simulink model "modell_kalman"  (R2013a)
settings: Solver=ode45  SolverMode=SingleTasking  StartTime=0.0  StopTime=10.0  RelTol=1e-3
values from neighbouring files (symbols this model uses):
  A = [0 1 0 0; d3 0 0 0;0 0 0 1; c3 0 0 0]    [startModell.m]
  B = [0 ; d1; 0 ; c1]    [startModell.m]
  beobachterNull = [0;0;0;0]    [startModell.m]
  C = [1 0 0 0; 0 0 1 0]    [startModell.m]
  K = lqr(A,B,Q_ctrl,R_ctrl)    [startModell.m]
  modellNull = [10/180*pi;0;0;0]    [startModell.m]
  P0 = diag([100,100,1,1])    [startModell.m]
  Q = eye(4)    [startModell.m]
  R = diag([10, 10])    [startModell.m]
  Rinv = inv(R)    [startModell.m]
undefined symbols (not defined in the file or in its folder): Filter, Kalman, library
libraries: simulink x1
settings Model: Creator=wall  LastModifiedBy=timoe
settings DataIOCC: SignalLoggingSaveFormat=ModelDataLogs
settings OptimizationCC: BlockReduction=off  BooleanDataType=off
settings DebuggingCC: SaveWithParameterizedLinksMsg=none  SignalResolutionControl=TryResolveAllWithWarning  SolverPrmCheckMsg=none  MultiTaskDSMMsg=warning  MultiTaskCondExecSysMsg=none  StrictBusMsg=None
settings HardwareCC: TargetUnknown=on
settings RTWCC: IncludeERTFirstTime=on

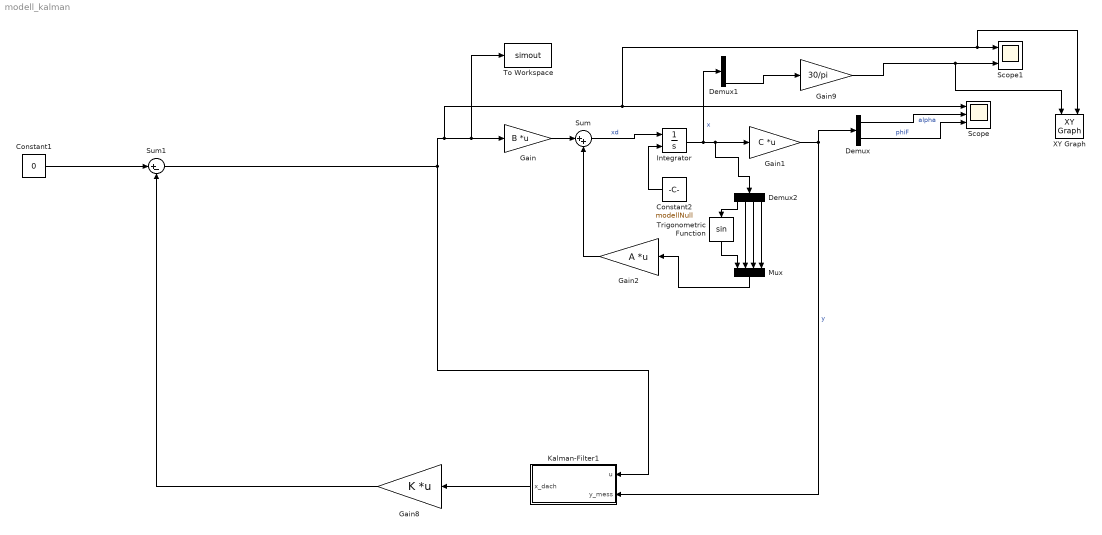
== system modell_kalman ==
  Constant1 : Constant  Value=0
  Constant2 : Constant  Value=modellNull
  Demux : Demux  Outputs=2
  Demux1 : Demux
  Demux2 : Demux
  Gain : Gain  Gain=B  Multiplication=Matrix(K*u) (u vector)
  Gain1 : Gain  Gain=C  Multiplication=Matrix(K*u) (u vector)
  Gain2 : Gain  Gain=A  Multiplication=Matrix(K*u) (u vector)
  Gain8 : Gain  Gain=K  Multiplication=Matrix(K*u) (u vector)
  Gain9 : Gain  Gain=30/pi
  Integrator : Integrator  InitialConditionSource=external
  Kalman-Filter1 : Subsystem  AncestorBlock=library/Kalman-Filter
  Mux : Mux
  Scope : Scope  NumInputPorts=3
      settings: YMin=-1~0.165806~-5  YMax=1~0.18326~5
  Scope1 : Scope  NumInputPorts=2
      settings: YMin=-5~-5  YMax=5~5
  Sum : Sum  Inputs=|++
  Sum1 : Sum  Inputs=|+-
  To Workspace : ToWorkspace  VariableName=simout  SampleTime=-1  SaveFormat=Timeseries
  Trigonometric Function : Trigonometry
  XY Graph : simulink/Sinks/XY Graph  xmin=-1  xmax=1  ymin=-1  ymax=1  st=-1
  wires:
  Integrator/1 -> Demux1/1, Demux2/1, Gain1/1  "x"
  Gain1/1 -> Kalman-Filter1/2(y_mess), Demux/1  "y"
  Gain2/1 -> Sum/2
  Sum/1 -> Integrator/1  "xd"
  Gain/1 -> Sum/1
  Gain8/1 -> Sum1/2
  Constant2/1 -> Integrator/2
  Sum1/1 -> Kalman-Filter1/1(u), XY Graph/2, Scope1/1, Scope/1, To Workspace/1, Gain/1
  Demux/1 -> Scope/2  "alpha"
  Demux/2 -> Scope/3  "phiF"
  Demux1/4 -> Gain9/1
  Gain9/1 -> XY Graph/1, Scope1/2
  Demux2/1 -> Trigonometric Function/1
  Trigonometric Function/1 -> Mux/1
  Demux2/2 -> Mux/2
  Demux2/3 -> Mux/3
  Demux2/4 -> Mux/4
  Mux/1 -> Gain2/1
  Kalman-Filter1/1(x_dach) -> Gain8/1
  Constant1/1 -> Sum1/1

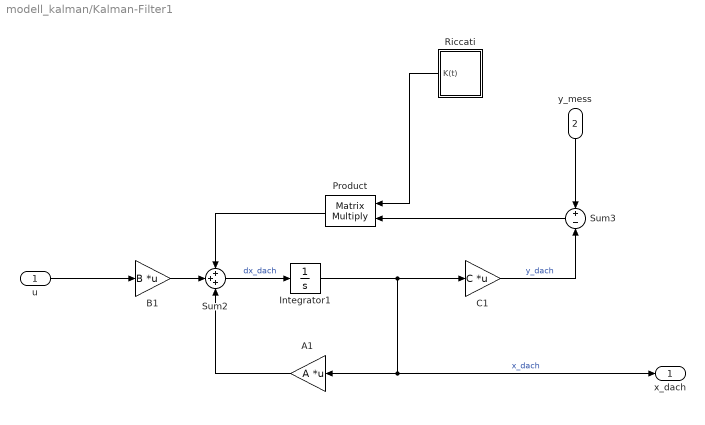
== system modell_kalman/Kalman-Filter1 ==
  u : Inport
  y_mess : Inport  Port=2
  A1 : Gain  Gain=A  Multiplication=Matrix(K*u)
  B1 : Gain  Gain=B  Multiplication=Matrix(K*u)
  C1 : Gain  Gain=C  Multiplication=Matrix(K*u)
  Integrator1 : Integrator  InitialCondition=beobachterNull
  Product : Product  Multiplication=Matrix(*)
  Riccati : Subsystem  AncestorBlock=library/Riccati
  Sum2 : Sum  Inputs=+++
  Sum3 : Sum  Inputs=+|-
  x_dach : Outport
  wires:
  Integrator1/1 -> x_dach/1, A1/1, C1/1  "x_dach"
  Sum2/1 -> Integrator1/1  "dx_dach"
  C1/1 -> Sum3/2  "y_dach"
  A1/1 -> Sum2/3
  B1/1 -> Sum2/2
  Product/1 -> Sum2/1
  u/1 -> B1/1
  y_mess/1 -> Sum3/1
  Sum3/1 -> Product/2
  Riccati/1(K(t)) -> Product/1

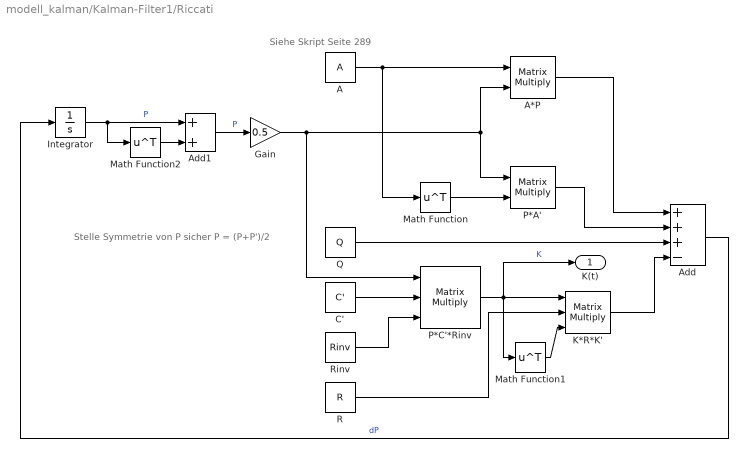
== system modell_kalman/Kalman-Filter1/Riccati ==
  note: Stelle Symmetrie von P sicher
      | P = (P+P')/2
  note: Siehe Skript Seite 289
  A : Constant  Value=A
  A*P : Product  Multiplication=Matrix(*)
  Add : Sum  Inputs=+++-
  Add1 : Sum
  C' : Constant  Value=C'
  Gain : Gain  Gain=0.5
  Integrator : Integrator  InitialCondition=P0
  K*R*K' : Product  Inputs=3  Multiplication=Matrix(*)
  Math Function : Math  Operator=transpose  SaturateOnIntegerOverflow=on
  Math Function1 : Math  Operator=transpose  SaturateOnIntegerOverflow=on
  Math Function2 : Math  Operator=transpose  SaturateOnIntegerOverflow=on
  P*A' : Product  Multiplication=Matrix(*)
  P*C'*Rinv : Product  Inputs=3  Multiplication=Matrix(*)
  Q : Constant  Value=Q
  R : Constant  Value=R
  Rinv : Constant  Value=Rinv
  K(t) : Outport
  wires:
  Gain/1 -> A*P/2, P*A'/1, P*C'*Rinv/1
  Math Function2/1 -> Add1/2
  Integrator/1 -> Add1/1, Math Function2/1  "P"
  Math Function1/1 -> K*R*K'/3
  A/1 -> Math Function/1, A*P/1
  Add1/1 -> Gain/1  "P"
  Math Function/1 -> P*A'/2
  C'/1 -> P*C'*Rinv/2
  P*C'*Rinv/1 -> Math Function1/1, K*R*K'/1, K(t)/1  "K"
  Rinv/1 -> P*C'*Rinv/3
  A*P/1 -> Add/1
  P*A'/1 -> Add/2
  Q/1 -> Add/3
  K*R*K'/1 -> Add/4
  Add/1 -> Integrator/1  "dP"
  R/1 -> K*R*K'/2
